simulink model "MANIP_PAC"  (R2022b)
settings: Solver=ode1  StartTime=0.0  StopTime=inf  FixedStep=25e-6  RelTol=1e-3
values from neighbouring files (symbols this model uses):
  C_buck = DeltaI_buck / (8 * fdec_buck * DeltaV_buck)    (= 1.32275132275e-06)    [BuckDesign_modinit.m]    (also in MANIP_BuckDesign_modinit.m = 1e-05)
  E_buck = 70    [BuckDesign_modinit.m]    (also in MANIP_BuckDesign_modinit.m)
  fdec_buck = 9e3    (= 9000)    [BuckDesign_modinit.m]    (also in MANIP_BuckDesign_modinit.m = 10000)
  Ki_buck = 3 / (t5_buck * K_buck)    (= 42.8571428571)    [BuckDesign_modinit.m]    (also in MANIP_BuckDesign_modinit.m)
  Kicalc_buck = Ppicalc_buck*Kpcalc_buck    [Buck_GM_PM_analysis.m]
  Kp_buck = tau_buck * Ki_buck    (= 0.00617283950617)    [BuckDesign_modinit.m]    (also in MANIP_BuckDesign_modinit.m = 0.00571428571429)
  Kpcalc_buck = 0.1    [Buck_GM_PM_analysis.m]
  L_boost = alphaMR_boost * E_boost / (DeltaI_boost * fdec_boost)    (= 0.00833333333333)    [BoostDesign_modinit.m]
  L_buck = (1 - alphaMR_buck) * alphaMR_buck * E_buck / (DeltaI_buck * fdec_buck)    (= 0.00648148148148)    [BuckDesign_modinit.m]    (also in MANIP_BuckDesign_modinit.m = 0.003)
  RealData = 1    [FullSystemPAC_init.m]    (also in MANIP_FULLSYSTEM.m)
  Rl_buck = 0    [BuckDesign_modinit.m]    (also in MANIP_BuckDesign_modinit.m)
  Rs_buck = Vnom_buck/1    (= 45)    [BuckDesign_modinit.m]    (also in Buck_GM_PM_analysis.m = (1/(2*epsfirst_buck))*sqrt(L_buck/C_buck); MANIP_BuckDesign_modinit.m = 22.5)
undefined symbols (not defined in the file or in its folder): Humusoft, L, MF624, Rl
libraries: sldrtlib x10, spsSeriesRLCBranchLib x3, spsVoltageMeasurementLib x3, spsCurrentMeasurementLib x2, simulink x2, spsDCVoltageSourceLib x1, spsDiodeLib x1, spsMosfetLib x1, pid_lib x1, spsControlledCurrentSourceLib x1, spsFuelCellStackLib x1, slpidlib x1
settings Model: SimulationMode=external  Creator=val thorens  LastModifiedBy=Etudiants
settings SolverCC: AlgebraicLoopSolver=TrustRegion
settings DataIOCC: ReturnWorkspaceOutputs=off
settings DebuggingCC: UnconnectedInputMsg=warning  UnconnectedOutputMsg=warning  UnconnectedLineMsg=warning  SFMachineParentedDataDiag=warning  ArithmeticOperatorsInVariantConditions=warning
settings HardwareCC: ProdBitPerLong=64  ProdHWDeviceType=Intel->x86-64 (Linux 64)
settings ModelReferenceCC: EnableRefExpFcnMdlSchedulingChecks=on
settings SFSimCC: CustomCodeUndefinedFunction=UseInterfaceOnly
settings RTWCC: Description=Simulink Desktop Real-Time  SystemTargetFile=sldrt.tlc  TemplateMakefile=sldrt.tmf  RTWCompilerOptimization=on  DLArmComputeVersion=19.05
settings CodeAppCC: MaxIdLength=95
settings SimulinkDesktopRealTimeCC: TargetLibSuffix=_sldrt.a  TargetPreCompLibLocation=D:\Program Files\MATLAB\R2022b\toolbox\sldrt\lib\win64  ParMdlRefBuildCompliant=on

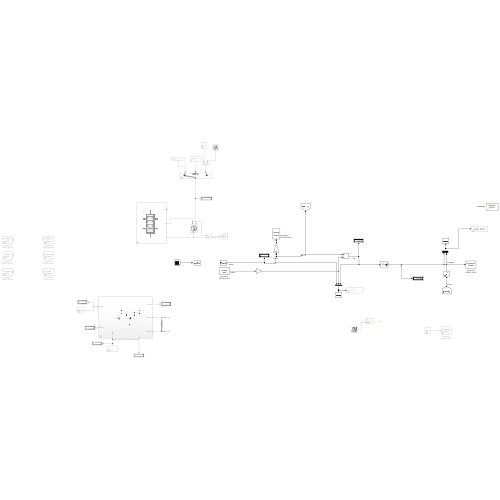
[thumbnail: Simulink's stored preview of the top-level diagram]
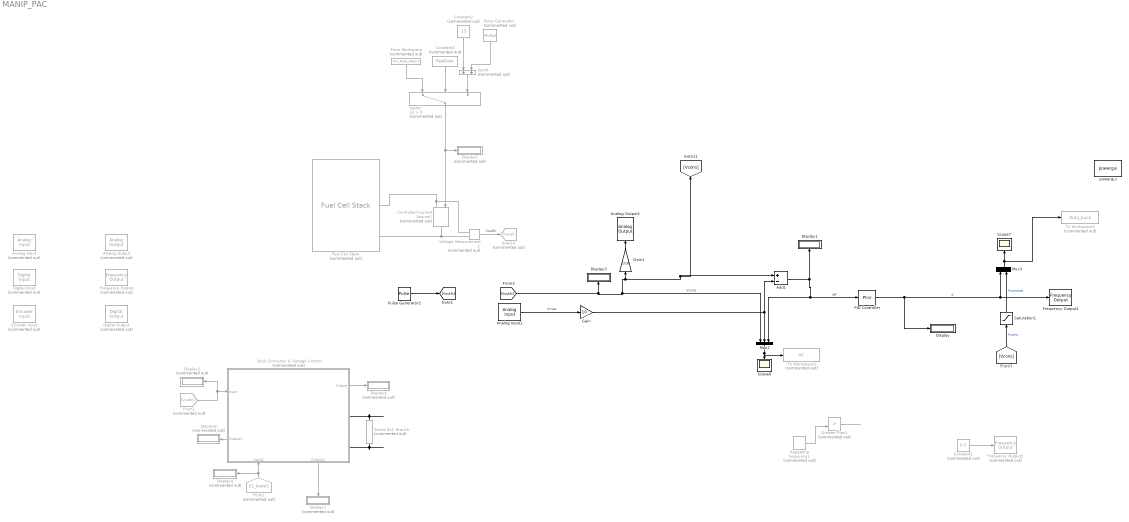
== system MANIP_PAC ==
  Add1 : Sum  Inputs=+-
  Analog Input : sldrtlib/Analog Input  Commented=on  SampleTime=-1  MaxMissedTicks=10  ShowMissedTicks=off  YieldWhenWaiting=off  DrvName=Humusoft/MF624  DrvAddress=4294967295  DrvOptions=585  Channels=1:4  RangeMode=1  VoltRange=1  DataType=1
      settings: AttributesFormatString=Humusoft\nMF624 [auto]
  Analog Input1 : sldrtlib/Analog Input  SampleTime=-1  MaxMissedTicks=10  ShowMissedTicks=off  YieldWhenWaiting=off  DrvName=Humusoft/MF624  DrvAddress=4294967295  DrvOptions=585  Channels=1  RangeMode=1  VoltRange=1  DataType=1
      settings: AttributesFormatString=Humusoft\nMF624 [auto]
  Analog Output : sldrtlib/Analog Output  Commented=on  SampleTime=-1  MaxMissedTicks=10  ShowMissedTicks=off  YieldWhenWaiting=off  DrvName=Humusoft/MF624  DrvAddress=4294967295  DrvOptions=585  Channels=1:4  RangeMode=1  VoltRange=1  InitialValue=0  FinalValue=0
      settings: AttributesFormatString=Humusoft\nMF624 [auto]
  Analog Output1 : sldrtlib/Analog Output  SampleTime=-1  MaxMissedTicks=10  ShowMissedTicks=off  YieldWhenWaiting=off  DrvName=Humusoft/MF624  DrvAddress=4294967295  DrvOptions=585  Channels=1  RangeMode=1  VoltRange=1  InitialValue=0  FinalValue=0
      settings: AttributesFormatString=Humusoft\nMF624 [auto]
  Buck Converter & Voltage Control : Subsystem  Commented=on
      settings: PortSchema="{\"entries\":[{\"content\":{\"sides\":[{\"content\":{\"connectorIds\":[\"In1\",\"Out3\"]},\"type\":\"ConnectorPlacement.EquallySpacedRectSide\",\"uuid\":\"253fbb6d-d91b-4b53-935c-694843fbf71e\"},{\"content\":{\"connectorIds\":[\"Out1\",\"RConn1\",\"RConn2\"],\"side\":\"RIGHT\"},\"type\":\"ConnectorPlacement.EquallySpacedRectSide\",\"uuid\":\"8dcd7ba1-263b-46b4-b8db-cd225d7ae698\"},{\"content\":{\"connectorIds\":[],\"side\":\"TOP\"},\"type\":\"ConnectorPlacement.EquallySpacedRectSide\",\"uuid\":\"1cdaf65b-d572-4b23-b30d-e9980adb48ec\"},{\"content\":{\"connectorIds\":[\"In2\",\"Out2\"],\"side\":\"BOTTOM\"},\"type\":\"ConnectorPlacement.EquallySpacedRectSide\",\"uuid\":\"ec595735-129f-488e-a889-595cc94a4f95\"}]},\"type\":\"ConnectorPlacement.EquallySpacedConnector\",\"uuid\":\"9cfd1eb3-dd0a-47bd-9e7c-3d98a8e839e7\"}],\"packageUris\":[\"http://schema.mathworks.com/mf0/Connector/R2020b\"],\"version\":\"1.0\"}"
  Constant1 : Constant  Commented=on  Value=0.5
  Constant2 : Constant  Commented=on  Value=15
  Constant3 : Constant  Commented=on  Value=RealData
  Controlled Current Source2 : spsControlledCurrentSourceLib/Controlled Current Source  Commented=on  Initialize=on  Source_Type=AC  Amplitude=0  Phase=0  Frequency=0  Measurements=None
  Digital Input : sldrtlib/Digital Input  Commented=on  SampleTime=-1  MaxMissedTicks=10  ShowMissedTicks=off  YieldWhenWaiting=off  DrvName=Humusoft/MF624  DrvAddress=4294967295  DrvOptions=585  Channels=1:8  BitMode=1  DataType=1
      settings: AttributesFormatString=Humusoft\nMF624 [auto]
  Digital Output : sldrtlib/Digital Output  Commented=on  SampleTime=-1  MaxMissedTicks=10  ShowMissedTicks=off  YieldWhenWaiting=off  DrvName=Humusoft/MF624  DrvAddress=4294967295  DrvOptions=585  Channels=1:4  BitMode=1  InitialValue=0  FinalValue=0
      settings: AttributesFormatString=Humusoft\nMF624 [auto]
  Display : Display
  Display1 : Display
  Display{2,4..5,7..9} (6 alike) : Display  Commented=on
  Display3 : Display
  Encoder Input : sldrtlib/Encoder Input  Commented=on  SampleTime=-1  MaxMissedTicks=10  ShowMissedTicks=off  YieldWhenWaiting=off  DrvName=Humusoft/MF624  DrvAddress=4294967295  DrvOptions=585  Channels=1  QuadMode=3  IndexPulse=3  InputFilter=Inf  DataType=1
      settings: AttributesFormatString=Humusoft\nMF624 [auto]
  Frequency Output : sldrtlib/Frequency Output  Commented=on  SampleTime=-1  MaxMissedTicks=10  ShowMissedTicks=off  YieldWhenWaiting=off  DrvName=Humusoft/MF624  DrvAddress=4294967295  DrvOptions=585  Channels=1:4  FrequencySource=1  Frequency=20000  FrequencyFinalValue=[]  DutySource=2  Duty=0.5  DutyFinalValue=0.5
      settings: AttributesFormatString=Humusoft\nMF624 [auto]
  Frequency Output1 : sldrtlib/Frequency Output  SampleTime=-1  MaxMissedTicks=10  ShowMissedTicks=off  YieldWhenWaiting=off  DrvName=Humusoft/MF624  DrvAddress=4294967295  DrvOptions=585  Channels=1  FrequencySource=1  Frequency=fdec_buck  FrequencyFinalValue=[]  DutySource=2  Duty=0.5  DutyFinalValue=0.5
      settings: AttributesFormatString=Humusoft\nMF624 [auto]
  Frequency Output2 : sldrtlib/Frequency Output  Commented=on  SampleTime=-1  MaxMissedTicks=10  ShowMissedTicks=off  YieldWhenWaiting=off  DrvName=Humusoft/MF624  DrvAddress=4294967295  DrvOptions=585  Channels=1  FrequencySource=1  Frequency=10000  FrequencyFinalValue=[]  DutySource=2  Duty=0.5  DutyFinalValue=0.5
      settings: AttributesFormatString=Humusoft\nMF624 [auto]
  From Workspace : FromWorkspace  Commented=on  VariableName=IFC_Real_Matrix  OutputAfterFinalValue=Holding final value
  From1 : From  Commented=on  GotoTag=Voutfc
  From2 : From  Commented=on  GotoTag=IL_boost  TagVisibility=global
  Fuel Cell Stack : spsFuelCellStackLib/Fuel Cell Stack  Commented=on  PresetModel=PEMFC - 6 kW - 45 Vdc  FcType=Proton Exchange Membrane (PEM)  Detailed=Detailed  Eoc=[65,63]  NomVI=[133.3,45]  EndVI=[225,37]  Nc=65  n=55  TOp=65  AirFr=300  SuppPress=[1.5,1]  Comp=[99.95,21,1]  SignX=off  SignY=off  FlowRateH2=off  FlowRateAir=off  SystemTemp=off  SystemPH2=off  SystemPAir=off  FCDyn=on  FC_tau=0.5  Peak_O2=80  V_Under=10
  Gain : Gain  Gain=10
  Gain1 : Gain  Gain=1/10
  Goto10 : Goto  Commented=on  GotoTag=Voutfc
  GreaterThan1 : RelationalOperator  Commented=on  Operator=>  OutDataTypeStr=boolean  RndMeth=Simplest  InputSameDT=off
  Mux2 : Mux  Inputs=3
  Mux3 : Mux  Inputs=2
  PID Controller : slpidlib/PID Controller  Controller=PI  Form=Parallel  TimeDomain=Continuous-time  UseExternalTs=off  SampleTime=-1  IntegratorMethod=Forward Euler  FilterMethod=Forward Euler  ControllerParametersSource=internal  P=Kpcalc_buck  I=Kicalc_buck  UseKiTs=off  D=0  N=100  UseFilter=on  TunerSelectOption=Transfer Function Based (PID Tuner App)  InitialConditionSource=internal  InitialConditionForIntegrator=0  InitialConditionForFilter=0  DifferentiatorICPrevScaledInput=0  ExternalReset=none  TrackingMode=off  Kt=1  LimitOutput=on  SatLimitsSource=internal  UpperSaturationLimit=1  LowerSaturationLimit=0  LinearizeAsGain=on  AntiWindupMode=clamping  Kb=1  LimitIntegrator=off  UpperIntegratorSaturationLimit=inf  LowerIntegratorSaturationLimit=-inf  POutMin=[]  POutMax=[]  IOutMin=[]  IOutMax=[]  DOutMin=[]  DOutMax=[]  NOutMin=[]  NOutMax=[]  SumOutMin=[]  SumOutMax=[]  SaturationOutMin=[]  SaturationOutMax=[]  PParamMin=[]  PParamMax=[]  IParamMin=[]  IParamMax=[]  DParamMin=[]  DParamMax=[]  NParamMin=[]  NParamMax=[]  KbParamMin=[]  KbParamMax=[]  KtParamMin=[]  KtParamMax=[]  KbOutMin=[]  KbOutMax=[]  KtOutMin=[]  KtOutMax=[]  IntegratorOutMin=[]  IntegratorOutMax=[]  FilterOutMin=[]  FilterOutMax=[]  SumI1OutMin=[]  SumI1OutMax=[]  SumI2OutMin=[]  SumI2OutMax=[]  SumI3OutMin=[]  SumI3OutMax=[]  SumI4OutMin=[]  SumI4OutMax=[]  SumDOutMin=[]  SumDOutMax=[]  DifferentiatorOutMin=[]  DifferentiatorOutMax=[]  FilterDiffOutCoefMin=[]  FilterDiffOutCoefMax=[]  ReciprocalOutMin=[]  ReciprocalOutMax=[]  SumDenOutMin=[]  SumDenOutMax=[]  SumNumOutMin=[]  SumNumOutMax=[]  DivideOutMin=[]  DivideOutMax=[]  UdiffTsProdOutMin=[]  UdiffTsProdOutMax=[]  NTsProdOutMin=[]  NTsProdOutMax=[]  UintegralTsProdOutMin=[]  UintegralTsProdOutMax=[]  UngainTsProdOutMin=[]  UngainTsProdOutMax=[]  ClampingZeroOutDataTypeStr=Inherit: Inherit via back propagation  ClampingZeroOutMin=[]  ClampingZeroOutMax=[]  FilterDenConstantOutDataTypeStr=Inherit: Inherit via back propagation  FilterDenConstantOutMin=[]  FilterDenConstantOutMax=[]  PCopyOutDataTypeStr=Inherit: Inherit via back propagation  PCopyOutMin=[]  PCopyOutMax=[]  NCopyOutDataTypeStr=Inherit: Inherit via back propagation  NCopyOutMin=[]  NCopyOutMax=[]  IntegratorContinuousStateAttributes=''  IntegratorStateMustResolveToSignalObject=off  IntegratorRTWStateStorageClass=Auto  FilterContinuousStateAttributes=''  FilterStateMustResolveToSignalObject=off  FilterRTWStateStorageClass=Auto  ParallelPVariant=InternalParameters  IdealPVariant=Disabled  IVariant=InternalParameters  DVariant=Disabled  IntegratorVariant=Continuous  SatVariant=Enabled  AWVariant=ContClampingParallel  PCopyVariant=Disabled  TRVariant=Disabled  FdbkBlocksVariant=Forward  IdealPFdbkVariant=Disabled  SatFdbkVariant=Disabled  DerivativeFilterVariant=Disabled  NVariant=Disabled  NCopyVariant=Disabled_SignalSpec  FilterICVariant=Disabled  IntegratorICVariant=InternalICs  ExternalResetVariant=Disabled  TRSumVariant=Passthrough  SumFdbkVariant=Disabled  SumVariant=Sum_PI  TsampFilterVariant=InternalTs  TsampNgainVariant=Passthrough  TsampIntegralVariant=Passthrough  ExternalSaturationOutDataTypeStr=Inherit: Same as second input
  Pulse Generator : DiscretePulseGenerator  Commented=on  PulseType=Time based  Period=100e-3  PulseWidth=50
  Pulse Generator2 : DiscretePulseGenerator  PulseType=Time based  Amplitude=55  Period=100e-3  PulseWidth=50
  Repeating Sequence1 : simulink/Sources/Repeating Sequence  Commented=on  rep_seq_t=[0 1/fdec_buck]  rep_seq_y=[0 1]
  Saturation1 : Saturate  UpperLimit=1  LowerLimit=0
  Scope6 : Scope
  Scope7 : Scope
  Series RLC Branch : spsSeriesRLCBranchLib/Series RLC Branch  Commented=on  LConnTagsString=__new0  RConnTagsString=__new0  BranchType=R  Resistance=Rs_buck  Inductance=L_boost  SetiL0=on  InitialCurrent=0  Capacitance=1e-6  Setx0=off  InitialVoltage=0  Measurements=None
  Sum3 : Sum  Commented=on
  Switch : Switch  Commented=on  Criteria=u2 > Threshold  SaturateOnIntegerOverflow=off  InputSameDT=off
  To Workspace2 : ToWorkspace  Commented=on  VariableName=VC  SaveFormat=Structure With Time  SampleTime=-1
  To Workspace3 : ToWorkspace  Commented=on  VariableName=Duty_buck  SaveFormat=Structure With Time  SampleTime=-1
  Voltage Measurement2 : spsVoltageMeasurementLib/Voltage Measurement  Commented=on  PhasorSimulation=off  OutputType=Complex  PSBequivalent=0
  powergui : spspowerguiLib/powergui  Priority=1  SimulationMode=Discrete  SampleTime=50e-6  frequency=60  Iterations=50  frequencyindice=0  Pbase=100e6  ErrMax=1e-4  UnitsV=kV  UnitsW=MW  buscounter=0  FunctionMessages=off  echomessages=off  EnableUseOfTLC=off  CurrentSourceSwitches=off  DisableSnubberDevices=on  DisableRonSwitches=on  DisableVfSwitches=on  DisplayEquations=off  AutomaticDiscreteSolvers=off  SolverType=Tustin  Interpol=off  ExternalGateDelay=off  methode=off  Ts=0  x0status=blocks  SPID=on  SwTol=0  HookPort=off  NonlinearTolerance=1e-4  nMaxIteration=100  ContinueOnMaxIteration=off  RestoreLinks=warning  ResistiveCurrentMeasurement=off  Frange=[0:2:500]  Ylog=off  Xlog=on  ShowGrid=off  save=off  variable=ZData  structure=0  ZoomFFT=off  StartTime=0.0  cycles=1  DisplayStyle=1  fundamental=60  FreqAxis=off  MaxFrequency=1000  frequencyindicesteady=1  RmsSteady=1  display=off
  wires:
  Buck Converter & Voltage Control/2(Output2) -> Display7/1
  From1/1 -> Display2/1, Buck Converter & Voltage Control/1(Input)
  From2/1 -> Display4/1, Buck Converter & Voltage Control/2(Input1)
  Voltage Measurement2/1 -> Goto10/1  "Voutfc"
  Buck Converter & Voltage Control/1(Output) -> Display9/1
  Switch/1 -> Display5/1, Controlled Current Source2/1
  Buck Converter & Voltage Control/3(Output1) -> Display8/1
  PID Controller/1 -> Display/1, Frequency Output1/1, Mux3/1  "d"
  Saturation1/1 -> Mux3/2  "Vconssat"
  [Voutfc] -> Gain1/1, [Vcons], Add1/1, Mux2/1, Display3/1  "Vcons"
  Analog Input1/1 -> Gain/1  "Vmes"
  Mux3/1 -> Scope7/1, To Workspace3/1
  Add1/1 -> PID Controller/1, Mux2/3, Display1/1  "dif"
  Mux2/1 -> To Workspace2/1, Scope6/1
  [Vcons] -> Saturation1/1  "Vcons"
  Repeating Sequence1/1 -> GreaterThan1/2
  GreaterThan1/1 -> ?
  Constant1/1 -> Frequency Output2/1
  Gain1/1 -> Analog Output1/1
  Pulse Generator2/1 -> [Voutfc]
  Gain/1 -> Add1/2, Mux2/2
  Pulse Generator/1 -> Sum3/2
  Constant2/1 -> Sum3/1
  From Workspace/1 -> Switch/1
  Sum3/1 -> Switch/3
  Constant3/1 -> Switch/2
  connections:
  Voltage Measurement2/LConn2 -- Controlled Current Source2/RConn1 -- Fuel Cell Stack/RConn2
  Buck Converter & Voltage Control/RConn2 -- Series RLC Branch/RConn1
  Voltage Measurement2/LConn1 -- Controlled Current Source2/LConn1 -- Fuel Cell Stack/RConn1
  Buck Converter & Voltage Control/RConn1 -- Series RLC Branch/LConn1

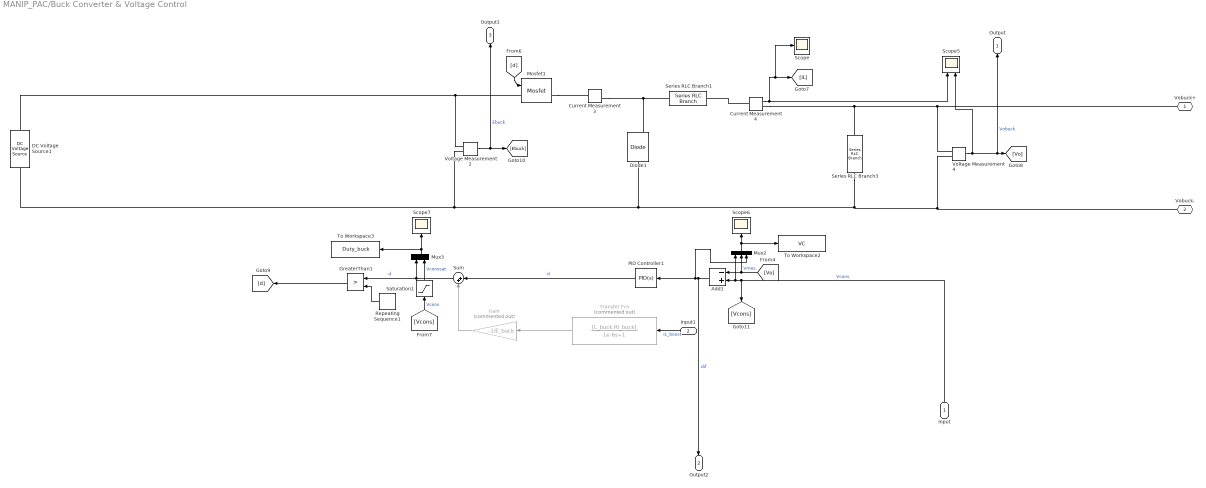
== system MANIP_PAC/Buck Converter & Voltage Control ==
  Input : Inport
  Input1 : Inport  Port=2
  Add1 : Sum  Inputs=-+
  Current Measurement3 : spsCurrentMeasurementLib/Current Measurement  PhasorSimulation=off  OutputType=Complex  PSBequivalent=0
  Current Measurement4 : spsCurrentMeasurementLib/Current Measurement  PhasorSimulation=off  OutputType=Complex  PSBequivalent=0
  DC Voltage Source1 : spsDCVoltageSourceLib/DC Voltage Source  Amplitude=E_buck  Measurements=None
  Diode1 : spsDiodeLib/Diode  Ron=0.000001  Lon=0  Vf=0  IC=0  UseSnubber=off  Rs=500  Cs=250e-9  Measurements=on
  Gain : Gain  Commented=on  Gain=-1/E_buck
  GreaterThan1 : RelationalOperator  Operator=>  OutDataTypeStr=boolean  RndMeth=Simplest  InputSameDT=off
  Mosfet1 : spsMosfetLib/Mosfet  Ron=0.01  Lon=0  Rd=0.01  Vfd=0  IC=0  Rs=1e5  Cs=inf  Measurements=on
  Mux2 : Mux  Inputs=3
  Mux3 : Mux  Inputs=2
  PID Controller1 : pid_lib/PID Controller  Controller=PID  Form=Parallel  TimeDomain=Continuous-time  UseExternalTs=off  SampleTime=-1  IntegratorMethod=Forward Euler  ControllerParametersSource=internal  P=Kp_buck  I=Ki_buck  D=0  N=100  UseFilter=on  TunerSelectOption=Transfer Function Based (PID Tuner App)  InitialConditionSource=internal  InitialConditionForIntegrator=0  InitialConditionForFilter=0  DifferentiatorICPrevScaledInput=0  ExternalReset=none  TrackingMode=off  Kt=1  LimitOutput=off  SatLimitsSource=internal  UpperSaturationLimit=inf  LowerSaturationLimit=-inf  LinearizeAsGain=on  AntiWindupMode=none  Kb=1  POutMin=[]  POutMax=[]  IOutMin=[]  IOutMax=[]  DOutMin=[]  DOutMax=[]  NOutMin=[]  NOutMax=[]  SumOutMin=[]  SumOutMax=[]  SaturationOutMin=[]  SaturationOutMax=[]  PParamMin=[]  PParamMax=[]  IParamMin=[]  IParamMax=[]  DParamMin=[]  DParamMax=[]  NParamMin=[]  NParamMax=[]  KbParamMin=[]  KbParamMax=[]  KtParamMin=[]  KtParamMax=[]  KbOutMin=[]  KbOutMax=[]  KtOutMin=[]  KtOutMax=[]  IntegratorOutMin=[]  IntegratorOutMax=[]  FilterOutMin=[]  FilterOutMax=[]  SumI1OutMin=[]  SumI1OutMax=[]  SumI2OutMin=[]  SumI2OutMax=[]  SumI3OutMin=[]  SumI3OutMax=[]  SumI4OutMin=[]  SumI4OutMax=[]  SumDOutMin=[]  SumDOutMax=[]  DifferentiatorOutMin=[]  DifferentiatorOutMax=[]  FilterDiffOutCoefMin=[]  FilterDiffOutCoefMax=[]  ReciprocalOutMin=[]  ReciprocalOutMax=[]  SumDenOutMin=[]  SumDenOutMax=[]  SumNumOutMin=[]  SumNumOutMax=[]  DivideOutMin=[]  DivideOutMax=[]  UdiffTsProdOutMin=[]  UdiffTsProdOutMax=[]  NTsProdOutMin=[]  NTsProdOutMax=[]  UintegralTsProdOutMin=[]  UintegralTsProdOutMax=[]  UngainTsProdOutMin=[]  UngainTsProdOutMax=[]  IntegratorContinuousStateAttributes=''  IntegratorStateMustResolveToSignalObject=off  IntegratorRTWStateStorageClass=Auto  FilterContinuousStateAttributes=''  FilterStateMustResolveToSignalObject=off  FilterRTWStateStorageClass=Auto  ParallelPVariant=InternalParameters  IdealPVariant=Disabled  IVariant=InternalParameters  DVariant=InternalParameters  IntegratorVariant=Continuous  SatVariant=Disabled  AWVariant=Passthrough  PCopyVariant=Disabled  TRVariant=Disabled  FdbkBlocksVariant=Forward  IdealPFdbkVariant=Disabled  SatFdbkVariant=Disabled  DerivativeFilterVariant=ContFilter  NVariant=InternalParameters  NCopyVariant=Disabled  FilterICVariant=InternalICsFilter  IntegratorICVariant=InternalICs  ExternalResetVariant=Disabled  TRSumVariant=Passthrough  SumFdbkVariant=Disabled  SumVariant=Sum_PID  TsampFilterVariant=InternalTs  TsampNgainVariant=Passthrough  TsampIntegralVariant=Disabled_SignalSpec  ExternalSaturationOutDataTypeStr=Inherit: Same as second input
  Repeating Sequence1 : simulink/Sources/Repeating Sequence  rep_seq_t=[0 1/fdec_buck]  rep_seq_y=[0 1]
  Saturation1 : Saturate  UpperLimit=1  LowerLimit=0
  Scope : Scope
  Scope5 : Scope  NumInputPorts=2
  Scope6 : Scope
  Scope7 : Scope
  Series RLC Branch1 : spsSeriesRLCBranchLib/Series RLC Branch  LConnTagsString=__new0  RConnTagsString=__new0  BranchType=RL  Resistance=Rl_buck  Inductance=L_buck  SetiL0=on  InitialCurrent=0  Capacitance=1e-6  Setx0=off  InitialVoltage=0  Measurements=None
  Series RLC Branch3 : spsSeriesRLCBranchLib/Series RLC Branch  LConnTagsString=__new0  RConnTagsString=__new0  BranchType=C  Resistance=Rl  Inductance=L  SetiL0=on  InitialCurrent=0  Capacitance=C_buck  Setx0=off  InitialVoltage=0  Measurements=None
  Sum : Sum  Inputs=|++
  To Workspace2 : ToWorkspace  VariableName=VC  SaveFormat=Timeseries  SampleTime=-1
  To Workspace3 : ToWorkspace  VariableName=Duty_buck  SaveFormat=Timeseries  SampleTime=-1
  Transfer Fcn : TransferFcn  Commented=on  Numerator=[L_buck Rl_buck]  Denominator=[1e-6 1]
  Voltage Measurement2 : spsVoltageMeasurementLib/Voltage Measurement  PhasorSimulation=off  OutputType=Complex  PSBequivalent=0
  Voltage Measurement4 : spsVoltageMeasurementLib/Voltage Measurement  PhasorSimulation=off  OutputType=Complex  PSBequivalent=0
  Vobuck+ : PMIOPort  Side=Right
  Vobuck- : PMIOPort  Port=2  Side=Right
  Output : Outport
  Output2 : Outport  Port=2
  Output1 : Outport  Port=3
  wires:
  Input/1 -> [Vcons], Mux2/1, Add1/2  "Vcons"
  [d] -> Mosfet1/1
  Mux3/1 -> To Workspace3/1, Scope7/1
  [Vo] -> Mux2/2, Add1/1  "Vmes"
  GreaterThan1/1 -> [d]
  Current Measurement4/1 -> Scope/1, [IL], Scope5/1
  Repeating Sequence1/1 -> GreaterThan1/2
  Add1/1 -> Output2/1, PID Controller1/1, Mux2/3  "dif"
  Sum/1 -> GreaterThan1/1, Mux3/1  "d"
  [Vcons] -> Saturation1/1  "Vcons"
  Voltage Measurement4/1 -> Scope5/2, Output/1, [Vo]  "Vobuck"
  Saturation1/1 -> Mux3/2  "Vconssat"
  Mux2/1 -> To Workspace2/1, Scope6/1
  Voltage Measurement2/1 -> Output1/1, [Ebuck]  "Ebuck"
  Input1/1 -> Transfer Fcn/1  "IL_boost"
  Transfer Fcn/1 -> Gain/1
  Gain/1 -> Sum/2
  PID Controller1/1 -> Sum/1  "d"
  connections:
  Diode1/LConn1 -- Vobuck-/RConn1 -- Voltage Measurement4/LConn2 -- Series RLC Branch3/LConn1 -- DC Voltage Source1/LConn1 -- Voltage Measurement2/LConn2
  Series RLC Branch1/RConn1 -- Current Measurement3/RConn1 -- Diode1/RConn1
  Mosfet1/LConn1 -- DC Voltage Source1/RConn1 -- Voltage Measurement2/LConn1
  Voltage Measurement4/LConn1 -- Vobuck+/RConn1 -- Current Measurement4/RConn1 -- Series RLC Branch3/RConn1
  Current Measurement4/LConn1 -- Series RLC Branch1/LConn1
  Mosfet1/RConn1 -- Current Measurement3/LConn1
